simulink model "questao2b"  (Simulink 3.00)
settings: Solver=ode45  StartTime=0.0  StopTime=10  RelTol=1e-3
libraries: simulink3 x1

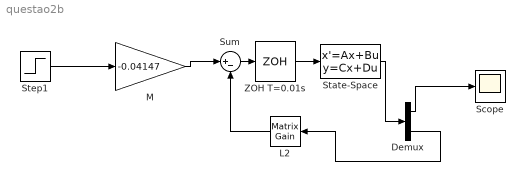
== system questao2b ==
  Demux : Demux  Outputs=2
  L2 : simulink3/Math/Matrix Gain  Orientation=left  K="[131.6205  555.7873   24.1488]"
  M : Gain  Gain=-0.04147  SaturateOnIntegerOverflow=on
  Scope : Scope
      settings: TimeRange=auto  YMin=-1  YMax=1  SaveToWorkspace=off  SaveName=ScopeData
  State-Space : StateSpace  A=[0 1 0 ;5.75 23.75 1; -2 0 1 ]  B=[0; 0 ;1]  C=[1 0 1;eye(3,3)]  D=[0;0;0;0]  X0=0
  Step1 : Step  Time=0  Before=0  After=1  SampleTime=0
  Sum : Sum  Inputs=|+-  SaturateOnIntegerOverflow=on
  ZOH T=0.01s : ZeroOrderHold  SampleTime=0.25
  wires:
  M/1 -> Sum/1
  Step1/1 -> M/1
  L2/1 -> Sum/2
  Sum/1 -> ZOH T=0.01s/1
  ZOH T=0.01s/1 -> State-Space/1
  Demux/1 -> Scope/1
  State-Space/1 -> Demux/1
  Demux/2 -> L2/1
